simulink model "adjoint"  (Simulink 7.7)
settings: Solver=ode45  StartTime=0.0  StopTime=10.0  RelTol=1e-3
settings Model: Creator=spu  LastModifiedBy=mestan

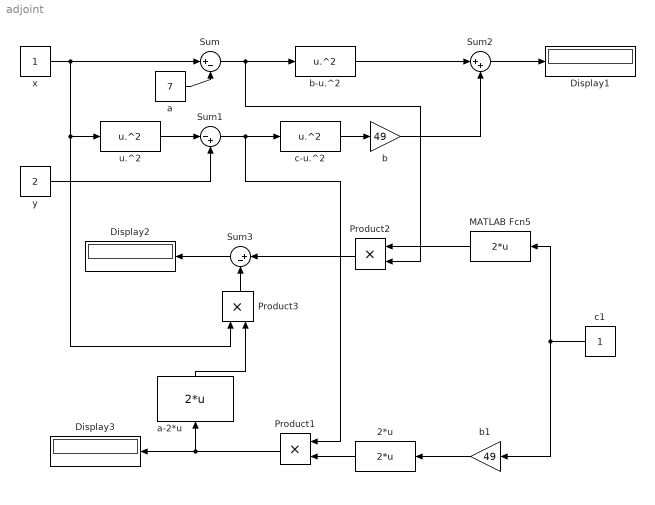
== system adjoint ==
  2*u : MATLABFcn  MATLABFcn=2*u
  Display1 : Display
  Display2 : Display
  Display3 : Display
  MATLAB Fcn5 : MATLABFcn  MATLABFcn=2*u
  Product1 : Product  RndMeth=Zero
  Product2 : Product  RndMeth=Zero
  Product3 : Product  RndMeth=Zero
  Sum : Sum  Inputs=|+-
  Sum1 : Sum  Inputs=|-+
  Sum2 : Sum  Inputs=|++
  Sum3 : Sum  Inputs=|+-
  a : Constant  Value=7
  a-2*u : MATLABFcn  MATLABFcn=2*u
  b : Gain  Gain=49
  b-u.^2 : MATLABFcn  MATLABFcn=u.^2
  b1 : Gain  Gain=49
  c-u.^2 : MATLABFcn  MATLABFcn=u.^2
  c1 : Constant
  u.^2 : MATLABFcn  MATLABFcn=u.^2
  x : Constant
  y : Constant  Value=2
  wires:
  Sum/1 -> b-u.^2/1, Product2/2
  x/1 -> Sum/1, u.^2/1, Product3/1
  y/1 -> Sum1/2
  Sum1/1 -> Product1/1, c-u.^2/1
  c-u.^2/1 -> b/1
  b-u.^2/1 -> Sum2/1
  b/1 -> Sum2/2
  Sum2/1 -> Display1/1
  c1/1 -> b1/1, MATLAB Fcn5/1
  MATLAB Fcn5/1 -> Product2/1
  b1/1 -> 2*u/1
  2*u/1 -> Product1/2
  Product2/1 -> Sum3/1
  Product1/1 -> Display3/1, a-2*u/1
  a-2*u/1 -> Product3/2
  Product3/1 -> Sum3/2
  Sum3/1 -> Display2/1
  a/1 -> Sum/2
  u.^2/1 -> Sum1/1
